simulink model "ELM_tictactoe_V2"  (R2021b)
settings: Solver=VariableStepAuto  StartTime=0.0  StopTime=inf  RelTol=1e-3
(part 2 of 136)

== system ELM_tictactoe_V2/Subsystem/Player Switcher a4 ==
  Key : Inport
  Switcher : Inport  Port=2
  AND 1 : MATLAB Function  TreatAsAtomicUnit=on
  Demultiplexer : Subsystem
      settings: PortSchema="{\"entries\":[{\"content\":{\"sides\":[{\"content\":{\"connectorIds\":[\"In1\"]},\"type\":\"ConnectorPlacement.EquallySpacedRectSide\",\"uuid\":\"6ccd7be5-9453-443a-8992-4f3046a94d81\"},{\"content\":{\"connectorIds\":[\"Out1\",\"Out2\"],\"side\":\"RIGHT\"},\"type\":\"ConnectorPlacement.EquallySpacedRectSide\",\"uuid\":\"9e3b2918-337b-479e-a737-e198b459be29\"},{\"content\":{\"connectorIds\":[],\"side\":\"TOP\"},\"type\":\"ConnectorPlacement.EquallySpacedRectSide\",\"uuid\":\"03b37edf-716a-49b3-8681-b476b437a461\"},{\"content\":{\"connectorIds\":[\"In2\"],\"side\":\"BOTTOM\"},\"type\":\"ConnectorPlacement.EquallySpacedRectSide\",\"uuid\":\"022ab476-2e55-4fe4-b85e-58af71f15e71\"}]},\"type\":\"ConnectorPlacement.EquallySpacedConnector\",\"uuid\":\"5541166b-b010-45a8-a1ab-2639d21d22e7\"}],\"packageUris\":[\"http://schema.mathworks.com/mf0/Connector/R2020b\"],\"version\":\"1.0\"}"
  Dlatch : Subsystem
  NOT : MATLAB Function  TreatAsAtomicUnit=on
  Unit Delay : UnitDelay  SampleTime=-1  HasFrameUpgradeWarning=on
  Unit Delay1 : UnitDelay  SampleTime=-1  HasFrameUpgradeWarning=on
  Unit Delay2 : UnitDelay  SampleTime=-1  HasFrameUpgradeWarning=on
  XOR5 : MATLAB Function  TreatAsAtomicUnit=on
  A : Outport
  B : Outport  Port=2
  wires:
  Key/1 -> Demultiplexer/1(Input), AND 1/1(input_a)
  Dlatch/1(Q) -> Demultiplexer/2(c)
  Demultiplexer/1(out0) -> XOR5/1(input_a), A/1
  Demultiplexer/2(out1) -> B/1, XOR5/2(input_b)
  Switcher/1 -> Dlatch/2(D)
  AND 1/1(output) -> Dlatch/1(Clock)  "o1"
  XOR5/1(output) -> NOT/1(input_a)  "o2"
  NOT/1(output) -> Unit Delay/1  "t1"
  Unit Delay/1 -> Unit Delay1/1
  Unit Delay1/1 -> Unit Delay2/1
  Unit Delay2/1 -> AND 1/2(input_b)

== system ELM_tictactoe_V2/Subsystem/Player Switcher a5 ==
  Key : Inport
  Switcher : Inport  Port=2
  AND 1 : MATLAB Function  TreatAsAtomicUnit=on
  Demultiplexer : Subsystem
      settings: PortSchema="{\"entries\":[{\"content\":{\"sides\":[{\"content\":{\"connectorIds\":[\"In1\"]},\"type\":\"ConnectorPlacement.EquallySpacedRectSide\",\"uuid\":\"6ccd7be5-9453-443a-8992-4f3046a94d81\"},{\"content\":{\"connectorIds\":[\"Out1\",\"Out2\"],\"side\":\"RIGHT\"},\"type\":\"ConnectorPlacement.EquallySpacedRectSide\",\"uuid\":\"9e3b2918-337b-479e-a737-e198b459be29\"},{\"content\":{\"connectorIds\":[],\"side\":\"TOP\"},\"type\":\"ConnectorPlacement.EquallySpacedRectSide\",\"uuid\":\"03b37edf-716a-49b3-8681-b476b437a461\"},{\"content\":{\"connectorIds\":[\"In2\"],\"side\":\"BOTTOM\"},\"type\":\"ConnectorPlacement.EquallySpacedRectSide\",\"uuid\":\"022ab476-2e55-4fe4-b85e-58af71f15e71\"}]},\"type\":\"ConnectorPlacement.EquallySpacedConnector\",\"uuid\":\"5541166b-b010-45a8-a1ab-2639d21d22e7\"}],\"packageUris\":[\"http://schema.mathworks.com/mf0/Connector/R2020b\"],\"version\":\"1.0\"}"
  Dlatch : Subsystem
  NOT : MATLAB Function  TreatAsAtomicUnit=on
  Unit Delay : UnitDelay  SampleTime=-1  HasFrameUpgradeWarning=on
  Unit Delay1 : UnitDelay  SampleTime=-1  HasFrameUpgradeWarning=on
  Unit Delay2 : UnitDelay  SampleTime=-1  HasFrameUpgradeWarning=on
  XOR5 : MATLAB Function  TreatAsAtomicUnit=on
  A : Outport
  B : Outport  Port=2
  wires:
  Key/1 -> Demultiplexer/1(Input), AND 1/1(input_a)
  Dlatch/1(Q) -> Demultiplexer/2(c)
  Demultiplexer/1(out0) -> XOR5/1(input_a), A/1
  Demultiplexer/2(out1) -> B/1, XOR5/2(input_b)
  Switcher/1 -> Dlatch/2(D)
  AND 1/1(output) -> Dlatch/1(Clock)  "o1"
  XOR5/1(output) -> NOT/1(input_a)  "o2"
  NOT/1(output) -> Unit Delay/1  "t1"
  Unit Delay/1 -> Unit Delay1/1
  Unit Delay1/1 -> Unit Delay2/1
  Unit Delay2/1 -> AND 1/2(input_b)

== system ELM_tictactoe_V2/Subsystem/Player Switcher a6 ==
  Key : Inport
  Switcher : Inport  Port=2
  AND 1 : MATLAB Function  TreatAsAtomicUnit=on
  Demultiplexer : Subsystem
      settings: PortSchema="{\"entries\":[{\"content\":{\"sides\":[{\"content\":{\"connectorIds\":[\"In1\"]},\"type\":\"ConnectorPlacement.EquallySpacedRectSide\",\"uuid\":\"6ccd7be5-9453-443a-8992-4f3046a94d81\"},{\"content\":{\"connectorIds\":[\"Out1\",\"Out2\"],\"side\":\"RIGHT\"},\"type\":\"ConnectorPlacement.EquallySpacedRectSide\",\"uuid\":\"9e3b2918-337b-479e-a737-e198b459be29\"},{\"content\":{\"connectorIds\":[],\"side\":\"TOP\"},\"type\":\"ConnectorPlacement.EquallySpacedRectSide\",\"uuid\":\"03b37edf-716a-49b3-8681-b476b437a461\"},{\"content\":{\"connectorIds\":[\"In2\"],\"side\":\"BOTTOM\"},\"type\":\"ConnectorPlacement.EquallySpacedRectSide\",\"uuid\":\"022ab476-2e55-4fe4-b85e-58af71f15e71\"}]},\"type\":\"ConnectorPlacement.EquallySpacedConnector\",\"uuid\":\"5541166b-b010-45a8-a1ab-2639d21d22e7\"}],\"packageUris\":[\"http://schema.mathworks.com/mf0/Connector/R2020b\"],\"version\":\"1.0\"}"
  Dlatch : Subsystem
  NOT : MATLAB Function  TreatAsAtomicUnit=on
  Unit Delay : UnitDelay  SampleTime=-1  HasFrameUpgradeWarning=on
  Unit Delay1 : UnitDelay  SampleTime=-1  HasFrameUpgradeWarning=on
  Unit Delay2 : UnitDelay  SampleTime=-1  HasFrameUpgradeWarning=on
  XOR5 : MATLAB Function  TreatAsAtomicUnit=on
  A : Outport
  B : Outport  Port=2
  wires:
  Key/1 -> Demultiplexer/1(Input), AND 1/1(input_a)
  Dlatch/1(Q) -> Demultiplexer/2(c)
  Demultiplexer/1(out0) -> XOR5/1(input_a), A/1
  Demultiplexer/2(out1) -> B/1, XOR5/2(input_b)
  Switcher/1 -> Dlatch/2(D)
  AND 1/1(output) -> Dlatch/1(Clock)  "o1"
  XOR5/1(output) -> NOT/1(input_a)  "o2"
  NOT/1(output) -> Unit Delay/1  "t1"
  Unit Delay/1 -> Unit Delay1/1
  Unit Delay1/1 -> Unit Delay2/1
  Unit Delay2/1 -> AND 1/2(input_b)

== system ELM_tictactoe_V2/Subsystem/Player Switcher a7 ==
  Key : Inport
  Switcher : Inport  Port=2
  AND 1 : MATLAB Function  TreatAsAtomicUnit=on
  Demultiplexer : Subsystem
      settings: PortSchema="{\"entries\":[{\"content\":{\"sides\":[{\"content\":{\"connectorIds\":[\"In1\"]},\"type\":\"ConnectorPlacement.EquallySpacedRectSide\",\"uuid\":\"6ccd7be5-9453-443a-8992-4f3046a94d81\"},{\"content\":{\"connectorIds\":[\"Out1\",\"Out2\"],\"side\":\"RIGHT\"},\"type\":\"ConnectorPlacement.EquallySpacedRectSide\",\"uuid\":\"9e3b2918-337b-479e-a737-e198b459be29\"},{\"content\":{\"connectorIds\":[],\"side\":\"TOP\"},\"type\":\"ConnectorPlacement.EquallySpacedRectSide\",\"uuid\":\"03b37edf-716a-49b3-8681-b476b437a461\"},{\"content\":{\"connectorIds\":[\"In2\"],\"side\":\"BOTTOM\"},\"type\":\"ConnectorPlacement.EquallySpacedRectSide\",\"uuid\":\"022ab476-2e55-4fe4-b85e-58af71f15e71\"}]},\"type\":\"ConnectorPlacement.EquallySpacedConnector\",\"uuid\":\"5541166b-b010-45a8-a1ab-2639d21d22e7\"}],\"packageUris\":[\"http://schema.mathworks.com/mf0/Connector/R2020b\"],\"version\":\"1.0\"}"
  Dlatch : Subsystem
  NOT : MATLAB Function  TreatAsAtomicUnit=on
  Unit Delay : UnitDelay  SampleTime=-1  HasFrameUpgradeWarning=on
  Unit Delay1 : UnitDelay  SampleTime=-1  HasFrameUpgradeWarning=on
  Unit Delay2 : UnitDelay  SampleTime=-1  HasFrameUpgradeWarning=on
  XOR5 : MATLAB Function  TreatAsAtomicUnit=on
  A : Outport
  B : Outport  Port=2
  wires:
  Key/1 -> Demultiplexer/1(Input), AND 1/1(input_a)
  Dlatch/1(Q) -> Demultiplexer/2(c)
  Demultiplexer/1(out0) -> XOR5/1(input_a), A/1
  Demultiplexer/2(out1) -> B/1, XOR5/2(input_b)
  Switcher/1 -> Dlatch/2(D)
  AND 1/1(output) -> Dlatch/1(Clock)  "o1"
  XOR5/1(output) -> NOT/1(input_a)  "o2"
  NOT/1(output) -> Unit Delay/1  "t1"
  Unit Delay/1 -> Unit Delay1/1
  Unit Delay1/1 -> Unit Delay2/1
  Unit Delay2/1 -> AND 1/2(input_b)

== system ELM_tictactoe_V2/Subsystem/Player Switcher a8 ==
  Key : Inport
  Switcher : Inport  Port=2
  AND 1 : MATLAB Function  TreatAsAtomicUnit=on
  Demultiplexer : Subsystem
      settings: PortSchema="{\"entries\":[{\"content\":{\"sides\":[{\"content\":{\"connectorIds\":[\"In1\"]},\"type\":\"ConnectorPlacement.EquallySpacedRectSide\",\"uuid\":\"6ccd7be5-9453-443a-8992-4f3046a94d81\"},{\"content\":{\"connectorIds\":[\"Out1\",\"Out2\"],\"side\":\"RIGHT\"},\"type\":\"ConnectorPlacement.EquallySpacedRectSide\",\"uuid\":\"9e3b2918-337b-479e-a737-e198b459be29\"},{\"content\":{\"connectorIds\":[],\"side\":\"TOP\"},\"type\":\"ConnectorPlacement.EquallySpacedRectSide\",\"uuid\":\"03b37edf-716a-49b3-8681-b476b437a461\"},{\"content\":{\"connectorIds\":[\"In2\"],\"side\":\"BOTTOM\"},\"type\":\"ConnectorPlacement.EquallySpacedRectSide\",\"uuid\":\"022ab476-2e55-4fe4-b85e-58af71f15e71\"}]},\"type\":\"ConnectorPlacement.EquallySpacedConnector\",\"uuid\":\"5541166b-b010-45a8-a1ab-2639d21d22e7\"}],\"packageUris\":[\"http://schema.mathworks.com/mf0/Connector/R2020b\"],\"version\":\"1.0\"}"
  Dlatch : Subsystem
  NOT : MATLAB Function  TreatAsAtomicUnit=on
  Unit Delay : UnitDelay  SampleTime=-1  HasFrameUpgradeWarning=on
  Unit Delay1 : UnitDelay  SampleTime=-1  HasFrameUpgradeWarning=on
  Unit Delay2 : UnitDelay  SampleTime=-1  HasFrameUpgradeWarning=on
  XOR5 : MATLAB Function  TreatAsAtomicUnit=on
  A : Outport
  B : Outport  Port=2
  wires:
  Key/1 -> Demultiplexer/1(Input), AND 1/1(input_a)
  Dlatch/1(Q) -> Demultiplexer/2(c)
  Demultiplexer/1(out0) -> XOR5/1(input_a), A/1
  Demultiplexer/2(out1) -> B/1, XOR5/2(input_b)
  Switcher/1 -> Dlatch/2(D)
  AND 1/1(output) -> Dlatch/1(Clock)  "o1"
  XOR5/1(output) -> NOT/1(input_a)  "o2"
  NOT/1(output) -> Unit Delay/1  "t1"
  Unit Delay/1 -> Unit Delay1/1
  Unit Delay1/1 -> Unit Delay2/1
  Unit Delay2/1 -> AND 1/2(input_b)

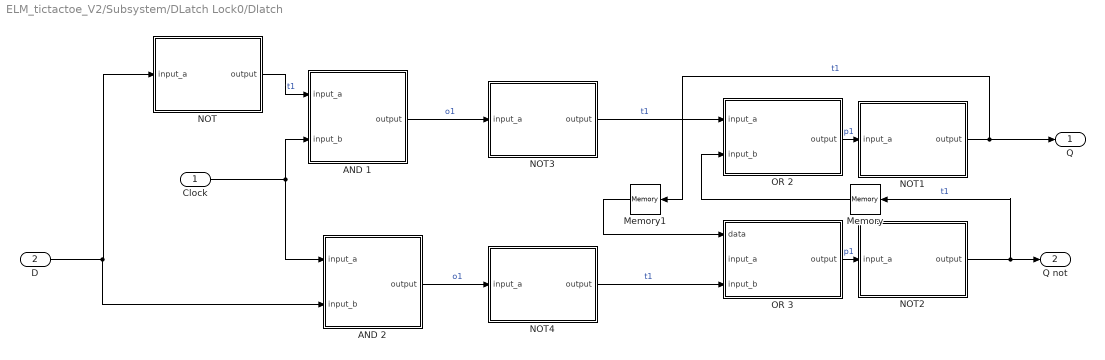
== system ELM_tictactoe_V2/Subsystem/DLatch Lock0/Dlatch ==
  Clock : Inport
  D : Inport  Port=2
  AND 1 : MATLAB Function  TreatAsAtomicUnit=on
  AND 2 : MATLAB Function  TreatAsAtomicUnit=on
  Memory : Memory
  Memory1 : Memory
  NOT : MATLAB Function  TreatAsAtomicUnit=on
  NOT1 : MATLAB Function  TreatAsAtomicUnit=on
  NOT2 : MATLAB Function  TreatAsAtomicUnit=on
  NOT3 : MATLAB Function  TreatAsAtomicUnit=on
  NOT4 : MATLAB Function  TreatAsAtomicUnit=on
  OR 2 : MATLAB Function  TreatAsAtomicUnit=on
  OR 3 : MATLAB Function  TreatAsAtomicUnit=on
  Q : Outport
  Q not : Outport  Port=2
  wires:
  D/1 -> AND 2/2(input_b), NOT/1(input_a)
  NOT/1(output) -> AND 1/1(input_a)  "t1"
  Clock/1 -> AND 1/2(input_b), AND 2/1(input_a)
  OR 2/1(output) -> NOT1/1(input_a)  "p1"
  OR 3/1(output) -> NOT2/1(input_a)  "p1"
  AND 2/1(output) -> NOT4/1(input_a)  "o1"
  NOT1/1(output) -> Q/1, Memory1/1  "t1"
  NOT2/1(output) -> Memory/1, Q not/1  "t1"
  AND 1/1(output) -> NOT3/1(input_a)  "o1"
  NOT3/1(output) -> OR 2/1(input_a)  "t1"
  NOT4/1(output) -> OR 3/3(input_b)  "t1"
  Memory/1 -> OR 2/2(input_b)
  Memory1/1 -> OR 3/1(data)

== system ELM_tictactoe_V2/Subsystem/DLatch Lock1/Dlatch ==
  D : Inport
  Clock : Inport  Port=2
  AND 1 : MATLAB Function  TreatAsAtomicUnit=on
  AND 2 : MATLAB Function  TreatAsAtomicUnit=on
  Memory : Memory  InitialCondition=1  LinearizeAsDelay=on
  Memory1 : Memory  LinearizeAsDelay=on
  NOT1 : MATLAB Function  TreatAsAtomicUnit=on
  NOT2 : MATLAB Function  TreatAsAtomicUnit=on
  NOT3 : MATLAB Function  TreatAsAtomicUnit=on
  OR 2 : MATLAB Function  TreatAsAtomicUnit=on
  OR 3 : MATLAB Function  TreatAsAtomicUnit=on
  Q : Outport
  Q not : Outport  Port=2
  wires:
  D/1 -> NOT3/1(input_a), AND 2/2(input_b)
  NOT3/1(output) -> AND 1/1(input_a)  "t1"
  Clock/1 -> AND 1/2(input_b), AND 2/1(input_a)
  OR 2/1(output) -> NOT1/1(input_a)  "p1"
  OR 3/1(output) -> NOT2/1(input_a)  "p1"
  AND 2/1(output) -> OR 3/2(input_b)  "o1"
  NOT1/1(output) -> Memory1/1, Q/1  "t1"
  NOT2/1(output) -> Memory/1, Q not/1  "t1"
  AND 1/1(output) -> OR 2/1(input_a)  "t1"
  Memory/1 -> OR 2/2(input_b)
  Memory1/1 -> OR 3/1(input_a)

== system ELM_tictactoe_V2/Subsystem/DLatch Lock2/Dlatch ==
  D : Inport
  Clock : Inport  Port=2
  AND 1 : MATLAB Function  TreatAsAtomicUnit=on
  AND 2 : MATLAB Function  TreatAsAtomicUnit=on
  Memory : Memory  InitialCondition=1  LinearizeAsDelay=on
  Memory1 : Memory  LinearizeAsDelay=on
  NOT1 : MATLAB Function  TreatAsAtomicUnit=on
  NOT2 : MATLAB Function  TreatAsAtomicUnit=on
  NOT3 : MATLAB Function  TreatAsAtomicUnit=on
  OR 2 : MATLAB Function  TreatAsAtomicUnit=on
  OR 3 : MATLAB Function  TreatAsAtomicUnit=on
  Q : Outport
  Q not : Outport  Port=2
  wires:
  D/1 -> NOT3/1(input_a), AND 2/2(input_b)
  NOT3/1(output) -> AND 1/1(input_a)  "t1"
  Clock/1 -> AND 1/2(input_b), AND 2/1(input_a)
  OR 2/1(output) -> NOT1/1(input_a)  "p1"
  OR 3/1(output) -> NOT2/1(input_a)  "p1"
  AND 2/1(output) -> OR 3/2(input_b)  "o1"
  NOT1/1(output) -> Memory1/1, Q/1  "t1"
  NOT2/1(output) -> Memory/1, Q not/1  "t1"
  AND 1/1(output) -> OR 2/1(input_a)  "t1"
  Memory/1 -> OR 2/2(input_b)
  Memory1/1 -> OR 3/1(input_a)

== system ELM_tictactoe_V2/Subsystem/DLatch Lock3/Dlatch ==
  D : Inport
  Clock : Inport  Port=2
  AND 1 : MATLAB Function  TreatAsAtomicUnit=on
  AND 2 : MATLAB Function  TreatAsAtomicUnit=on
  Memory : Memory  InitialCondition=1  LinearizeAsDelay=on
  Memory1 : Memory  LinearizeAsDelay=on
  NOT1 : MATLAB Function  TreatAsAtomicUnit=on
  NOT2 : MATLAB Function  TreatAsAtomicUnit=on
  NOT3 : MATLAB Function  TreatAsAtomicUnit=on
  OR 2 : MATLAB Function  TreatAsAtomicUnit=on
  OR 3 : MATLAB Function  TreatAsAtomicUnit=on
  Q : Outport
  Q not : Outport  Port=2
  wires:
  D/1 -> NOT3/1(input_a), AND 2/2(input_b)
  NOT3/1(output) -> AND 1/1(input_a)  "t1"
  Clock/1 -> AND 1/2(input_b), AND 2/1(input_a)
  OR 2/1(output) -> NOT1/1(input_a)  "p1"
  OR 3/1(output) -> NOT2/1(input_a)  "p1"
  AND 2/1(output) -> OR 3/2(input_b)  "o1"
  NOT1/1(output) -> Memory1/1, Q/1  "t1"
  NOT2/1(output) -> Memory/1, Q not/1  "t1"
  AND 1/1(output) -> OR 2/1(input_a)  "t1"
  Memory/1 -> OR 2/2(input_b)
  Memory1/1 -> OR 3/1(input_a)

== system ELM_tictactoe_V2/Subsystem/DLatch Lock4/Dlatch ==
  D : Inport
  Clock : Inport  Port=2
  AND 1 : MATLAB Function  TreatAsAtomicUnit=on
  AND 2 : MATLAB Function  TreatAsAtomicUnit=on
  Memory : Memory  InitialCondition=1  LinearizeAsDelay=on
  Memory1 : Memory  LinearizeAsDelay=on
  NOT1 : MATLAB Function  TreatAsAtomicUnit=on
  NOT2 : MATLAB Function  TreatAsAtomicUnit=on
  NOT3 : MATLAB Function  TreatAsAtomicUnit=on
  OR 2 : MATLAB Function  TreatAsAtomicUnit=on
  OR 3 : MATLAB Function  TreatAsAtomicUnit=on
  Q : Outport
  Q not : Outport  Port=2
  wires:
  D/1 -> NOT3/1(input_a), AND 2/2(input_b)
  NOT3/1(output) -> AND 1/1(input_a)  "t1"
  Clock/1 -> AND 1/2(input_b), AND 2/1(input_a)
  OR 2/1(output) -> NOT1/1(input_a)  "p1"
  OR 3/1(output) -> NOT2/1(input_a)  "p1"
  AND 2/1(output) -> OR 3/2(input_b)  "o1"
  NOT1/1(output) -> Memory1/1, Q/1  "t1"
  NOT2/1(output) -> Memory/1, Q not/1  "t1"
  AND 1/1(output) -> OR 2/1(input_a)  "t1"
  Memory/1 -> OR 2/2(input_b)
  Memory1/1 -> OR 3/1(input_a)

== system ELM_tictactoe_V2/Subsystem/DLatch Lock5/Dlatch ==
  D : Inport
  Clock : Inport  Port=2
  AND 1 : MATLAB Function  TreatAsAtomicUnit=on
  AND 2 : MATLAB Function  TreatAsAtomicUnit=on
  Memory : Memory  InitialCondition=1  LinearizeAsDelay=on
  Memory1 : Memory  LinearizeAsDelay=on
  NOT1 : MATLAB Function  TreatAsAtomicUnit=on
  NOT2 : MATLAB Function  TreatAsAtomicUnit=on
  NOT3 : MATLAB Function  TreatAsAtomicUnit=on
  OR 2 : MATLAB Function  TreatAsAtomicUnit=on
  OR 3 : MATLAB Function  TreatAsAtomicUnit=on
  Q : Outport
  Q not : Outport  Port=2
  wires:
  D/1 -> NOT3/1(input_a), AND 2/2(input_b)
  NOT3/1(output) -> AND 1/1(input_a)  "t1"
  Clock/1 -> AND 1/2(input_b), AND 2/1(input_a)
  OR 2/1(output) -> NOT1/1(input_a)  "p1"
  OR 3/1(output) -> NOT2/1(input_a)  "p1"
  AND 2/1(output) -> OR 3/2(input_b)  "o1"
  NOT1/1(output) -> Memory1/1, Q/1  "t1"
  NOT2/1(output) -> Memory/1, Q not/1  "t1"
  AND 1/1(output) -> OR 2/1(input_a)  "t1"
  Memory/1 -> OR 2/2(input_b)
  Memory1/1 -> OR 3/1(input_a)

== system ELM_tictactoe_V2/Subsystem/DLatch Lock6/Dlatch ==
  D : Inport
  Clock : Inport  Port=2
  AND 1 : MATLAB Function  TreatAsAtomicUnit=on
  AND 2 : MATLAB Function  TreatAsAtomicUnit=on
  Memory : Memory  InitialCondition=1  LinearizeAsDelay=on
  Memory1 : Memory  LinearizeAsDelay=on
  NOT1 : MATLAB Function  TreatAsAtomicUnit=on
  NOT2 : MATLAB Function  TreatAsAtomicUnit=on
  NOT3 : MATLAB Function  TreatAsAtomicUnit=on
  OR 2 : MATLAB Function  TreatAsAtomicUnit=on
  OR 3 : MATLAB Function  TreatAsAtomicUnit=on
  Q : Outport
  Q not : Outport  Port=2
  wires:
  D/1 -> NOT3/1(input_a), AND 2/2(input_b)
  NOT3/1(output) -> AND 1/1(input_a)  "t1"
  Clock/1 -> AND 1/2(input_b), AND 2/1(input_a)
  OR 2/1(output) -> NOT1/1(input_a)  "p1"
  OR 3/1(output) -> NOT2/1(input_a)  "p1"
  AND 2/1(output) -> OR 3/2(input_b)  "o1"
  NOT1/1(output) -> Memory1/1, Q/1  "t1"
  NOT2/1(output) -> Memory/1, Q not/1  "t1"
  AND 1/1(output) -> OR 2/1(input_a)  "t1"
  Memory/1 -> OR 2/2(input_b)
  Memory1/1 -> OR 3/1(input_a)

== system ELM_tictactoe_V2/Subsystem/DLatch Lock7/Dlatch ==
  D : Inport
  Clock : Inport  Port=2
  AND 1 : MATLAB Function  TreatAsAtomicUnit=on
  AND 2 : MATLAB Function  TreatAsAtomicUnit=on
  Memory : Memory  InitialCondition=1  LinearizeAsDelay=on
  Memory1 : Memory  LinearizeAsDelay=on
  NOT1 : MATLAB Function  TreatAsAtomicUnit=on
  NOT2 : MATLAB Function  TreatAsAtomicUnit=on
  NOT3 : MATLAB Function  TreatAsAtomicUnit=on
  OR 2 : MATLAB Function  TreatAsAtomicUnit=on
  OR 3 : MATLAB Function  TreatAsAtomicUnit=on
  Q : Outport
  Q not : Outport  Port=2
  wires:
  D/1 -> NOT3/1(input_a), AND 2/2(input_b)
  NOT3/1(output) -> AND 1/1(input_a)  "t1"
  Clock/1 -> AND 1/2(input_b), AND 2/1(input_a)
  OR 2/1(output) -> NOT1/1(input_a)  "p1"
  OR 3/1(output) -> NOT2/1(input_a)  "p1"
  AND 2/1(output) -> OR 3/2(input_b)  "o1"
  NOT1/1(output) -> Memory1/1, Q/1  "t1"
  NOT2/1(output) -> Memory/1, Q not/1  "t1"
  AND 1/1(output) -> OR 2/1(input_a)  "t1"
  Memory/1 -> OR 2/2(input_b)
  Memory1/1 -> OR 3/1(input_a)

== system ELM_tictactoe_V2/Subsystem/DLatch Lock8/Dlatch ==
  D : Inport
  Clock : Inport  Port=2
  AND 1 : MATLAB Function  TreatAsAtomicUnit=on
  AND 2 : MATLAB Function  TreatAsAtomicUnit=on
  Memory : Memory  InitialCondition=1  LinearizeAsDelay=on
  Memory1 : Memory  LinearizeAsDelay=on
  NOT1 : MATLAB Function  TreatAsAtomicUnit=on
  NOT2 : MATLAB Function  TreatAsAtomicUnit=on
  NOT3 : MATLAB Function  TreatAsAtomicUnit=on
  OR 2 : MATLAB Function  TreatAsAtomicUnit=on
  OR 3 : MATLAB Function  TreatAsAtomicUnit=on
  Q : Outport
  Q not : Outport  Port=2
  wires:
  D/1 -> NOT3/1(input_a), AND 2/2(input_b)
  NOT3/1(output) -> AND 1/1(input_a)  "t1"
  Clock/1 -> AND 1/2(input_b), AND 2/1(input_a)
  OR 2/1(output) -> NOT1/1(input_a)  "p1"
  OR 3/1(output) -> NOT2/1(input_a)  "p1"
  AND 2/1(output) -> OR 3/2(input_b)  "o1"
  NOT1/1(output) -> Memory1/1, Q/1  "t1"
  NOT2/1(output) -> Memory/1, Q not/1  "t1"
  AND 1/1(output) -> OR 2/1(input_a)  "t1"
  Memory/1 -> OR 2/2(input_b)
  Memory1/1 -> OR 3/1(input_a)

== system ELM_tictactoe_V2/Subsystem/DLatch Lock9/Dlatch ==
  D : Inport
  Clock : Inport  Port=2
  AND 1 : MATLAB Function  TreatAsAtomicUnit=on
  AND 2 : MATLAB Function  TreatAsAtomicUnit=on
  Memory : Memory  InitialCondition=1  LinearizeAsDelay=on
  Memory1 : Memory  LinearizeAsDelay=on
  NOT1 : MATLAB Function  TreatAsAtomicUnit=on
  NOT2 : MATLAB Function  TreatAsAtomicUnit=on
  NOT3 : MATLAB Function  TreatAsAtomicUnit=on
  OR 2 : MATLAB Function  TreatAsAtomicUnit=on
  OR 3 : MATLAB Function  TreatAsAtomicUnit=on
  Q : Outport
  Q not : Outport  Port=2
  wires:
  D/1 -> NOT3/1(input_a), AND 2/2(input_b)
  NOT3/1(output) -> AND 1/1(input_a)  "t1"
  Clock/1 -> AND 1/2(input_b), AND 2/1(input_a)
  OR 2/1(output) -> NOT1/1(input_a)  "p1"
  OR 3/1(output) -> NOT2/1(input_a)  "p1"
  AND 2/1(output) -> OR 3/2(input_b)  "o1"
  NOT1/1(output) -> Memory1/1, Q/1  "t1"
  NOT2/1(output) -> Memory/1, Q not/1  "t1"
  AND 1/1(output) -> OR 2/1(input_a)  "t1"
  Memory/1 -> OR 2/2(input_b)
  Memory1/1 -> OR 3/1(input_a)

== system ELM_tictactoe_V2/Subsystem/Player Switcher a/Demultiplexer ==
  note: if problems switch outputs
  Input : Inport
  c : Inport  Port=2
  AND 1 : MATLAB Function  TreatAsAtomicUnit=on
  AND 2 : MATLAB Function  TreatAsAtomicUnit=on
  NOT : MATLAB Function  TreatAsAtomicUnit=on
  out0 : Outport
  out1 : Outport  Port=2
  wires:
  c/1 -> AND 1/2(input_b), NOT/1(input_a)
  AND 2/1(output) -> out0/1  "o1"
  AND 1/1(output) -> out1/1  "o1"
  Input/1 -> AND 1/1(input_a), AND 2/2(input_b)
  NOT/1(output) -> AND 2/1(input_a)  "t1"

== system ELM_tictactoe_V2/Subsystem/Player Switcher a/Dlatch ==
  Clock : Inport
  D : Inport  Port=2
  AND 1 : MATLAB Function  TreatAsAtomicUnit=on
  AND 2 : MATLAB Function  TreatAsAtomicUnit=on
  Memory : Memory  InitialCondition=1  LinearizeAsDelay=on
  Memory1 : Memory  LinearizeAsDelay=on
  NOT : MATLAB Function  TreatAsAtomicUnit=on
  NOT1 : MATLAB Function  TreatAsAtomicUnit=on
  NOT2 : MATLAB Function  TreatAsAtomicUnit=on
  OR 2 : MATLAB Function  TreatAsAtomicUnit=on
  OR 3 : MATLAB Function  TreatAsAtomicUnit=on
  Q : Outport
  Q not : Outport  Port=2
  wires:
  D/1 -> AND 2/2(input_b), NOT/1(input_a)
  NOT/1(output) -> AND 1/1(input_a)  "t1"
  Clock/1 -> AND 1/2(input_b), AND 2/1(input_a)
  OR 2/1(output) -> NOT1/1(input_a)  "p1"
  OR 3/1(output) -> NOT2/1(input_a)  "p1"
  AND 2/1(output) -> OR 3/2(input_b)  "o1"
  NOT1/1(output) -> Memory1/1, Q/1  "t1"
  NOT2/1(output) -> Memory/1, Q not/1  "t1"
  AND 1/1(output) -> OR 2/1(input_a)  "t1"
  Memory/1 -> OR 2/2(input_b)
  Memory1/1 -> OR 3/1(input_a)

== system ELM_tictactoe_V2/Subsystem/Player Switcher a1/Demultiplexer ==
  note: if problems switch outputs
  Input : Inport
  c : Inport  Port=2
  AND 1 : MATLAB Function  TreatAsAtomicUnit=on
  AND 2 : MATLAB Function  TreatAsAtomicUnit=on
  NOT : MATLAB Function  TreatAsAtomicUnit=on
  out0 : Outport
  out1 : Outport  Port=2
  wires:
  c/1 -> AND 1/2(input_b), NOT/1(input_a)
  AND 2/1(output) -> out0/1  "o1"
  AND 1/1(output) -> out1/1  "o1"
  Input/1 -> AND 1/1(input_a), AND 2/2(input_b)
  NOT/1(output) -> AND 2/1(input_a)  "t1"

== system ELM_tictactoe_V2/Subsystem/Player Switcher a1/Dlatch ==
  Clock : Inport
  D : Inport  Port=2
  AND 1 : MATLAB Function  TreatAsAtomicUnit=on
  AND 2 : MATLAB Function  TreatAsAtomicUnit=on
  Memory : Memory  InitialCondition=1  LinearizeAsDelay=on
  Memory1 : Memory  LinearizeAsDelay=on
  NOT : MATLAB Function  TreatAsAtomicUnit=on
  NOT1 : MATLAB Function  TreatAsAtomicUnit=on
  NOT2 : MATLAB Function  TreatAsAtomicUnit=on
  OR 2 : MATLAB Function  TreatAsAtomicUnit=on
  OR 3 : MATLAB Function  TreatAsAtomicUnit=on
  Q : Outport
  Q not : Outport  Port=2
  wires:
  D/1 -> AND 2/2(input_b), NOT/1(input_a)
  NOT/1(output) -> AND 1/1(input_a)  "t1"
  Clock/1 -> AND 1/2(input_b), AND 2/1(input_a)
  OR 2/1(output) -> NOT1/1(input_a)  "p1"
  OR 3/1(output) -> NOT2/1(input_a)  "p1"
  AND 2/1(output) -> OR 3/2(input_b)  "o1"
  NOT1/1(output) -> Memory1/1, Q/1  "t1"
  NOT2/1(output) -> Memory/1, Q not/1  "t1"
  AND 1/1(output) -> OR 2/1(input_a)  "t1"
  Memory/1 -> OR 2/2(input_b)
  Memory1/1 -> OR 3/1(input_a)

== system ELM_tictactoe_V2/Subsystem/Player Switcher a2/Demultiplexer ==
  note: if problems switch outputs
  Input : Inport
  c : Inport  Port=2
  AND 1 : MATLAB Function  TreatAsAtomicUnit=on
  AND 2 : MATLAB Function  TreatAsAtomicUnit=on
  NOT : MATLAB Function  TreatAsAtomicUnit=on
  out0 : Outport
  out1 : Outport  Port=2
  wires:
  c/1 -> AND 1/2(input_b), NOT/1(input_a)
  AND 2/1(output) -> out0/1  "o1"
  AND 1/1(output) -> out1/1  "o1"
  Input/1 -> AND 1/1(input_a), AND 2/2(input_b)
  NOT/1(output) -> AND 2/1(input_a)  "t1"

== system ELM_tictactoe_V2/Subsystem/Player Switcher a2/Dlatch ==
  Clock : Inport
  D : Inport  Port=2
  AND 1 : MATLAB Function  TreatAsAtomicUnit=on
  AND 2 : MATLAB Function  TreatAsAtomicUnit=on
  Memory : Memory  InitialCondition=1  LinearizeAsDelay=on
  Memory1 : Memory  LinearizeAsDelay=on
  NOT : MATLAB Function  TreatAsAtomicUnit=on
  NOT1 : MATLAB Function  TreatAsAtomicUnit=on
  NOT2 : MATLAB Function  TreatAsAtomicUnit=on
  OR 2 : MATLAB Function  TreatAsAtomicUnit=on
  OR 3 : MATLAB Function  TreatAsAtomicUnit=on
  Q : Outport
  Q not : Outport  Port=2
  wires:
  D/1 -> AND 2/2(input_b), NOT/1(input_a)
  NOT/1(output) -> AND 1/1(input_a)  "t1"
  Clock/1 -> AND 1/2(input_b), AND 2/1(input_a)
  OR 2/1(output) -> NOT1/1(input_a)  "p1"
  OR 3/1(output) -> NOT2/1(input_a)  "p1"
  AND 2/1(output) -> OR 3/2(input_b)  "o1"
  NOT1/1(output) -> Memory1/1, Q/1  "t1"
  NOT2/1(output) -> Memory/1, Q not/1  "t1"
  AND 1/1(output) -> OR 2/1(input_a)  "t1"
  Memory/1 -> OR 2/2(input_b)
  Memory1/1 -> OR 3/1(input_a)

== system ELM_tictactoe_V2/Subsystem/Player Switcher a3/Demultiplexer ==
  note: if problems switch outputs
  Input : Inport
  c : Inport  Port=2
  AND 1 : MATLAB Function  TreatAsAtomicUnit=on
  AND 2 : MATLAB Function  TreatAsAtomicUnit=on
  NOT : MATLAB Function  TreatAsAtomicUnit=on
  out0 : Outport
  out1 : Outport  Port=2
  wires:
  c/1 -> AND 1/2(input_b), NOT/1(input_a)
  AND 2/1(output) -> out0/1  "o1"
  AND 1/1(output) -> out1/1  "o1"
  Input/1 -> AND 1/1(input_a), AND 2/2(input_b)
  NOT/1(output) -> AND 2/1(input_a)  "t1"

== system ELM_tictactoe_V2/Subsystem/Player Switcher a3/Dlatch ==
  Clock : Inport
  D : Inport  Port=2
  AND 1 : MATLAB Function  TreatAsAtomicUnit=on
  AND 2 : MATLAB Function  TreatAsAtomicUnit=on
  Memory : Memory  InitialCondition=1  LinearizeAsDelay=on
  Memory1 : Memory  LinearizeAsDelay=on
  NOT : MATLAB Function  TreatAsAtomicUnit=on
  NOT1 : MATLAB Function  TreatAsAtomicUnit=on
  NOT2 : MATLAB Function  TreatAsAtomicUnit=on
  OR 2 : MATLAB Function  TreatAsAtomicUnit=on
  OR 3 : MATLAB Function  TreatAsAtomicUnit=on
  Q : Outport
  Q not : Outport  Port=2
  wires:
  D/1 -> AND 2/2(input_b), NOT/1(input_a)
  NOT/1(output) -> AND 1/1(input_a)  "t1"
  Clock/1 -> AND 1/2(input_b), AND 2/1(input_a)
  OR 2/1(output) -> NOT1/1(input_a)  "p1"
  OR 3/1(output) -> NOT2/1(input_a)  "p1"
  AND 2/1(output) -> OR 3/2(input_b)  "o1"
  NOT1/1(output) -> Memory1/1, Q/1  "t1"
  NOT2/1(output) -> Memory/1, Q not/1  "t1"
  AND 1/1(output) -> OR 2/1(input_a)  "t1"
  Memory/1 -> OR 2/2(input_b)
  Memory1/1 -> OR 3/1(input_a)

== system ELM_tictactoe_V2/Subsystem/Player Switcher a4/Demultiplexer ==
  note: if problems switch outputs
  Input : Inport
  c : Inport  Port=2
  AND 1 : MATLAB Function  TreatAsAtomicUnit=on
  AND 2 : MATLAB Function  TreatAsAtomicUnit=on
  NOT : MATLAB Function  TreatAsAtomicUnit=on
  out0 : Outport
  out1 : Outport  Port=2
  wires:
  c/1 -> AND 1/2(input_b), NOT/1(input_a)
  AND 2/1(output) -> out0/1  "o1"
  AND 1/1(output) -> out1/1  "o1"
  Input/1 -> AND 1/1(input_a), AND 2/2(input_b)
  NOT/1(output) -> AND 2/1(input_a)  "t1"

== system ELM_tictactoe_V2/Subsystem/Player Switcher a4/Dlatch ==
  Clock : Inport
  D : Inport  Port=2
  AND 1 : MATLAB Function  TreatAsAtomicUnit=on
  AND 2 : MATLAB Function  TreatAsAtomicUnit=on
  Memory : Memory  InitialCondition=1  LinearizeAsDelay=on
  Memory1 : Memory  LinearizeAsDelay=on
  NOT : MATLAB Function  TreatAsAtomicUnit=on
  NOT1 : MATLAB Function  TreatAsAtomicUnit=on
  NOT2 : MATLAB Function  TreatAsAtomicUnit=on
  OR 2 : MATLAB Function  TreatAsAtomicUnit=on
  OR 3 : MATLAB Function  TreatAsAtomicUnit=on
  Q : Outport
  Q not : Outport  Port=2
  wires:
  D/1 -> AND 2/2(input_b), NOT/1(input_a)
  NOT/1(output) -> AND 1/1(input_a)  "t1"
  Clock/1 -> AND 1/2(input_b), AND 2/1(input_a)
  OR 2/1(output) -> NOT1/1(input_a)  "p1"
  OR 3/1(output) -> NOT2/1(input_a)  "p1"
  AND 2/1(output) -> OR 3/2(input_b)  "o1"
  NOT1/1(output) -> Memory1/1, Q/1  "t1"
  NOT2/1(output) -> Memory/1, Q not/1  "t1"
  AND 1/1(output) -> OR 2/1(input_a)  "t1"
  Memory/1 -> OR 2/2(input_b)
  Memory1/1 -> OR 3/1(input_a)

== system ELM_tictactoe_V2/Subsystem/Player Switcher a5/Demultiplexer ==
  note: if problems switch outputs
  Input : Inport
  c : Inport  Port=2
  AND 1 : MATLAB Function  TreatAsAtomicUnit=on
  AND 2 : MATLAB Function  TreatAsAtomicUnit=on
  NOT : MATLAB Function  TreatAsAtomicUnit=on
  out0 : Outport
  out1 : Outport  Port=2
  wires:
  c/1 -> AND 1/2(input_b), NOT/1(input_a)
  AND 2/1(output) -> out0/1  "o1"
  AND 1/1(output) -> out1/1  "o1"
  Input/1 -> AND 1/1(input_a), AND 2/2(input_b)
  NOT/1(output) -> AND 2/1(input_a)  "t1"

== system ELM_tictactoe_V2/Subsystem/Player Switcher a5/Dlatch ==
  Clock : Inport
  D : Inport  Port=2
  AND 1 : MATLAB Function  TreatAsAtomicUnit=on
  AND 2 : MATLAB Function  TreatAsAtomicUnit=on
  Memory : Memory  InitialCondition=1  LinearizeAsDelay=on
  Memory1 : Memory  LinearizeAsDelay=on
  NOT : MATLAB Function  TreatAsAtomicUnit=on
  NOT1 : MATLAB Function  TreatAsAtomicUnit=on
  NOT2 : MATLAB Function  TreatAsAtomicUnit=on
  OR 2 : MATLAB Function  TreatAsAtomicUnit=on
  OR 3 : MATLAB Function  TreatAsAtomicUnit=on
  Q : Outport
  Q not : Outport  Port=2
  wires:
  D/1 -> AND 2/2(input_b), NOT/1(input_a)
  NOT/1(output) -> AND 1/1(input_a)  "t1"
  Clock/1 -> AND 1/2(input_b), AND 2/1(input_a)
  OR 2/1(output) -> NOT1/1(input_a)  "p1"
  OR 3/1(output) -> NOT2/1(input_a)  "p1"
  AND 2/1(output) -> OR 3/2(input_b)  "o1"
  NOT1/1(output) -> Memory1/1, Q/1  "t1"
  NOT2/1(output) -> Memory/1, Q not/1  "t1"
  AND 1/1(output) -> OR 2/1(input_a)  "t1"
  Memory/1 -> OR 2/2(input_b)
  Memory1/1 -> OR 3/1(input_a)

== system ELM_tictactoe_V2/Subsystem/Player Switcher a6/Demultiplexer ==
  note: if problems switch outputs
  Input : Inport
  c : Inport  Port=2
  AND 1 : MATLAB Function  TreatAsAtomicUnit=on
  AND 2 : MATLAB Function  TreatAsAtomicUnit=on
  NOT : MATLAB Function  TreatAsAtomicUnit=on
  out0 : Outport
  out1 : Outport  Port=2
  wires:
  c/1 -> AND 1/2(input_b), NOT/1(input_a)
  AND 2/1(output) -> out0/1  "o1"
  AND 1/1(output) -> out1/1  "o1"
  Input/1 -> AND 1/1(input_a), AND 2/2(input_b)
  NOT/1(output) -> AND 2/1(input_a)  "t1"

== system ELM_tictactoe_V2/Subsystem/Player Switcher a6/Dlatch ==
  Clock : Inport
  D : Inport  Port=2
  AND 1 : MATLAB Function  TreatAsAtomicUnit=on
  AND 2 : MATLAB Function  TreatAsAtomicUnit=on
  Memory : Memory  InitialCondition=1  LinearizeAsDelay=on
  Memory1 : Memory  LinearizeAsDelay=on
  NOT : MATLAB Function  TreatAsAtomicUnit=on
  NOT1 : MATLAB Function  TreatAsAtomicUnit=on
  NOT2 : MATLAB Function  TreatAsAtomicUnit=on
  OR 2 : MATLAB Function  TreatAsAtomicUnit=on
  OR 3 : MATLAB Function  TreatAsAtomicUnit=on
  Q : Outport
  Q not : Outport  Port=2
  wires:
  D/1 -> AND 2/2(input_b), NOT/1(input_a)
  NOT/1(output) -> AND 1/1(input_a)  "t1"
  Clock/1 -> AND 1/2(input_b), AND 2/1(input_a)
  OR 2/1(output) -> NOT1/1(input_a)  "p1"
  OR 3/1(output) -> NOT2/1(input_a)  "p1"
  AND 2/1(output) -> OR 3/2(input_b)  "o1"
  NOT1/1(output) -> Memory1/1, Q/1  "t1"
  NOT2/1(output) -> Memory/1, Q not/1  "t1"
  AND 1/1(output) -> OR 2/1(input_a)  "t1"
  Memory/1 -> OR 2/2(input_b)
  Memory1/1 -> OR 3/1(input_a)

== system ELM_tictactoe_V2/Subsystem/Player Switcher a7/Demultiplexer ==
  note: if problems switch outputs
  Input : Inport
  c : Inport  Port=2
  AND 1 : MATLAB Function  TreatAsAtomicUnit=on
  AND 2 : MATLAB Function  TreatAsAtomicUnit=on
  NOT : MATLAB Function  TreatAsAtomicUnit=on
  out0 : Outport
  out1 : Outport  Port=2
  wires:
  c/1 -> AND 1/2(input_b), NOT/1(input_a)
  AND 2/1(output) -> out0/1  "o1"
  AND 1/1(output) -> out1/1  "o1"
  Input/1 -> AND 1/1(input_a), AND 2/2(input_b)
  NOT/1(output) -> AND 2/1(input_a)  "t1"

== system ELM_tictactoe_V2/Subsystem/Player Switcher a7/Dlatch ==
  Clock : Inport
  D : Inport  Port=2
  AND 1 : MATLAB Function  TreatAsAtomicUnit=on
  AND 2 : MATLAB Function  TreatAsAtomicUnit=on
  Memory : Memory  InitialCondition=1  LinearizeAsDelay=on
  Memory1 : Memory  LinearizeAsDelay=on
  NOT : MATLAB Function  TreatAsAtomicUnit=on
  NOT1 : MATLAB Function  TreatAsAtomicUnit=on
  NOT2 : MATLAB Function  TreatAsAtomicUnit=on
  OR 2 : MATLAB Function  TreatAsAtomicUnit=on
  OR 3 : MATLAB Function  TreatAsAtomicUnit=on
  Q : Outport
  Q not : Outport  Port=2
  wires:
  D/1 -> AND 2/2(input_b), NOT/1(input_a)
  NOT/1(output) -> AND 1/1(input_a)  "t1"
  Clock/1 -> AND 1/2(input_b), AND 2/1(input_a)
  OR 2/1(output) -> NOT1/1(input_a)  "p1"
  OR 3/1(output) -> NOT2/1(input_a)  "p1"
  AND 2/1(output) -> OR 3/2(input_b)  "o1"
  NOT1/1(output) -> Memory1/1, Q/1  "t1"
  NOT2/1(output) -> Memory/1, Q not/1  "t1"
  AND 1/1(output) -> OR 2/1(input_a)  "t1"
  Memory/1 -> OR 2/2(input_b)
  Memory1/1 -> OR 3/1(input_a)

== system ELM_tictactoe_V2/Subsystem/Player Switcher a8/Demultiplexer ==
  note: if problems switch outputs
  Input : Inport
  c : Inport  Port=2
  AND 1 : MATLAB Function  TreatAsAtomicUnit=on
  AND 2 : MATLAB Function  TreatAsAtomicUnit=on
  NOT : MATLAB Function  TreatAsAtomicUnit=on
  out0 : Outport
  out1 : Outport  Port=2
  wires:
  c/1 -> AND 1/2(input_b), NOT/1(input_a)
  AND 2/1(output) -> out0/1  "o1"
  AND 1/1(output) -> out1/1  "o1"
  Input/1 -> AND 1/1(input_a), AND 2/2(input_b)
  NOT/1(output) -> AND 2/1(input_a)  "t1"

== system ELM_tictactoe_V2/Subsystem/Player Switcher a8/Dlatch ==
  Clock : Inport
  D : Inport  Port=2
  AND 1 : MATLAB Function  TreatAsAtomicUnit=on
  AND 2 : MATLAB Function  TreatAsAtomicUnit=on
  Memory : Memory  InitialCondition=1  LinearizeAsDelay=on
  Memory1 : Memory  LinearizeAsDelay=on
  NOT : MATLAB Function  TreatAsAtomicUnit=on
  NOT1 : MATLAB Function  TreatAsAtomicUnit=on
  NOT2 : MATLAB Function  TreatAsAtomicUnit=on
  OR 2 : MATLAB Function  TreatAsAtomicUnit=on
  OR 3 : MATLAB Function  TreatAsAtomicUnit=on
  Q : Outport
  Q not : Outport  Port=2
  wires:
  D/1 -> AND 2/2(input_b), NOT/1(input_a)
  NOT/1(output) -> AND 1/1(input_a)  "t1"
  Clock/1 -> AND 1/2(input_b), AND 2/1(input_a)
  OR 2/1(output) -> NOT1/1(input_a)  "p1"
  OR 3/1(output) -> NOT2/1(input_a)  "p1"
  AND 2/1(output) -> OR 3/2(input_b)  "o1"
  NOT1/1(output) -> Memory1/1, Q/1  "t1"
  NOT2/1(output) -> Memory/1, Q not/1  "t1"
  AND 1/1(output) -> OR 2/1(input_a)  "t1"
  Memory/1 -> OR 2/2(input_b)
  Memory1/1 -> OR 3/1(input_a)

== matlab function ELM_tictactoe_V2/Subsystem/Player Switcher a3/AND 1 ==
  data: input_a input; output output; input_b input
function output = ELM_AND_GATE(input_a,input_b)

W_in = [-20.4234998482374,-12.1406464752050;34.9662774645120,22.3048610747550;27.5135014076671,-11.8821136728163;43.3930560102998,29.1918291598582;11.6077007014000,-20.6506922893688;14.2726521436761,43.6692489761432;26.0464241886903,-9.68461191223183;28.5719086471357,-10.8625362969641;-44.8168664480278,-13.6630468269807;23.5832355674709,13.5178565205153;-0.595190155998191,32.6675264444015;-29.9910715366289,45.6368482533294;11.1109896755286,21.9724926010718;2.41096999999016,-30.8928020058105;-17.6380174262979,5.70411447112569;44.7963438180664,1.56617907096882;-20.6073071149438,-1.13858395595620;-20.9577988920251,5.42344400162102;-49.5887758676920,-6.17198415081061;-34.0672953155536,-23.4293882641728;42.0964373437748,2.08995994157947;16.0594842530402,-5.82742188618444;-24.1979673298498,20.0846357449426;14.1637955150501,-22.4093782451237;32.5019316440185,-47.7850742497659;5.65020748573521,-11.0558169220352;18.2860320074285,-13.5071921579294;-17.1338584251542,-0.289471368113610;79.8912249283554,-5.88289863046220;10.6167563438988,-21.6598424073464;-13.7120799496915,-25.7154131557099;29.4525761375705,-12.7340321868342;-52.3779403317386,48.4475929312710;-21.1053810203369,8.67400007274519;1.22993887326798,-3.70624692809957;-9.49856413179175,0.365690191879251;3.12900384491283,-0.904046456494743;7.50031956301589,12.3562905429823;6.43847488045511,39.2896929930343;30.9682913693970,-5.61260179380429;16.7208437458437,-8.93490027926457;9.16686338753494,56.7173561810963;0.0624559228070524,37.6697462339016;2.26330809713934,-31.5009505093967;-23.0049138108282,-41.5936241178010;-62.7614859944072,-28.5377598082390;-20.3656390340748,26.5074415703121;13.0862756695891,32.7324925017909;-14.8270753763793,-5.78908508095375;-36.7521730583284,9.86331038699916;30.7962679604583,-29.8559393603953;3.30373449393291,-10.5420304923620;-8.88117192704538,41.3303683202268;52.8999308566504,49.2318116154372;2.64158643963260,29.7777212516651;-31.9516412904338,66.0214783191805;25.7858271202722,-0.599436983789141;-33.1933459392193,-93.7843176189170;-21.9684124077570,-10.0769874165693;-46.2472363729114,-14.3156847131541;28.5206530919700,-37.9884661829570;-19.8272908012971,69.8206134424084;-60.3758844801787,-42.4986961801329;-48.0099240618389,43.2234111412034;36.9254540912872,-13.1099151080403;-5.68510756080214,-26.0976234853871;-8.11958271580063,13.3720867169582;-21.0633654435240,16.7354311467768;-57.1207020235893,35.5563977733588;-65.1929314913375,-21.9837655787721;-37.6217408807725,-20.6384038955951;84.2465567073162,27.1791826321299;39.8658260327592,-10.6410700792742;-26.7682286164832,-72.3620841457909;1.74228260500578,14.6987682407339;21.8314451872695,15.1545073222707;42.7734556804950,23.3053437107014;-52.3620474579486,-20.3070405291868;19.2066460686292,15.7282876188390;-28.1106773217216,43.0106924395391;4.34091817403331,-0.938947535803997;8.15815993778319,7.00469292746946;-8.95604207834383,-15.3998774409149;30.8017678895126,42.4660493858867;-17.2027808718314,-43.0309249568029;-21.9058944343869,7.63216437262147;-15.8982331214174,-87.8145268594438;-27.7880796216369,-62.1366554729360;-41.9872676071158,-37.0115089790813;-11.7876138344444,-18.6291455076347;-7.47108258146190,8.03099015819682;20.3031299554645,33.4991878115674;38.0367786645124,-45.9246778881033;-8.29756542801905,-18.7227382185443;-33.6772876877293,-8.13292522732060;1.23339911855664,24.2129095366567;19.4308341367927,-30.5938654997904;6.79504332625115,-12.8844642712938;4.09955943436103,-20.5529136861469;11.6474041405598,-10.2871769777538;-32.8559493774495,5.71941024997113;-13.3710644186996,-0.402235293952540;-55.3649370062477,9.90949896419729;10.3270944663458,-29.8206623734780;4.22237250760553,-15.4172531344176;-15.4388166937508,-38.9411634802937;-30.2422972307137,71.4956633189874;-12.9295495050203,-20.4110897033136;-48.0054796021967,-9.08675732421978;-25.6056200193537,3.17644033581957;30.6981662616174,61.6688203564539;-45.2662334936500,27.7915162166928;14.4139129010152,21.0677813690493;-53.2017685177607,-35.7644445241302;24.1028061148554,-5.04209787159278;40.7333655228055,-41.1553973407627;-43.5388328453299,10.8684050043691;-30.4708782776919,-7.55038729329319;20.0091647944412,-31.2798983911486;-1.19761713513697,34.5151579892012;-52.1267782097328,-54.7999948864971;-3.43666069424264,-26.5011615898042;-2.03310965759943,25.9285263561512;-26.0608455261549,-1.94358186102191;22.2739611789588,16.2564688893720;10.3975189569990,-50.9892153592224;-64.2056486613328,7.47116060246074;-15.5306111774140,-75.4292639210629;-14.4846452736577,50.1733276192943;0.0536610508167438,-3.27928990065061;-39.0545284067751,17.6636910104571;60.8120997091226,59.6641132793492;-4.18651394222449,33.4671448130509;-8.25243891799725,11.4486964692483;-25.9357479933522,-30.2822733916141;-27.3681458591677,0.342036135988558;6.97838101085754,8.20864206293599;3.03038466844881,-58.2632778760971;16.8993606770075,27.9108422231432;-27.0306341473338,-16.4765235366297;12.3646480910480,-27.9789983458528;-41.4985406489430,-13.0317554805855;-37.3791894534236,-8.50333619541164;-11.8982142980850,7.92441211996077;-9.72327330637509,12.1774956717125;15.9151700148394,20.6586769292605;41.4517412948654,-33.8120618698675;-39.2097412558798,-35.0917718016543;-1.36102370170649,-23.6649017506674;33.8944529438942,-33.8691869760874;-11.5688556677587,6.90628898547454;-0.278997796545284,-40.2141298570031;-13.7583283899933,13.1495187767439;-2.55425370337439,18.7363075473572;-39.4201451724125,32.9554924738448;36.7914506136300,-25.3543367232876;-12.7478218817958,47.9692398155069;10.2153628006544,9.87314562341864;-10.5614702168624,-13.0679362604975;20.8754008242970,6.54992052454898;-16.0458783309429,-40.5324064255838;30.3903700568314,9.34371987004970;-5.73837021567895,-25.6544990836216;15.4677589505125,-5.46693028001366;-47.3470681950565,-26.7624365219556;55.1855894325610,56.7414574276919;4.95842686431410,-35.6265373056285;29.7658408895663,6.11363001016659;-10.2831888009040,-22.1198355665407;10.0974051267114,26.9308351287914;-15.7852653064450,2.38949940621357;-50.5623081232901,9.59402907412139;-39.1366095708553,-11.7415086290372;12.7641711957722,-45.7962691570206;15.6936239614246,12.2595525827837;-21.3232661826075,-65.2199146482455;20.0508832545707,35.9684970232014;-19.7384288284593,15.6196390009822;-15.1826405246133,11.8802271472769;-6.40511792295145,-13.1342969543437;-0.907888672104065,19.9790797942738;-3.62858905372617,27.5934815700635;-10.2941327496090,-65.8643234916195;5.14557929572198,-15.0513081657779;46.3680947983112,-24.3541482668530;-8.64616721191304,-21.8697002119886;42.0890073145846,0.606048851138131;-2.06520021899472,-30.0471840716136;-21.7210791340497,-9.25588737795911;-30.1012999580862,-1.07385072967672;44.0154506521947,27.1629656743690;11.8497051934589,24.2944668413671;-9.16626772673761,-0.594061241792559;-3.30673632578662,47.9350979629852;38.6763561458939,-52.8725841883569;30.9713154780136,-29.3188547199508;25.2369382014317,-30.9360615257859;42.4411313477873,13.3429221299133;-5.93919430230613,5.47803671824044;42.5121640232097,4.00601476069030];

b1 = [-1.41578459326034;-2.82092899987627;59.0356966809787;1.95735210329088;42.1258073093999;-21.1530754048030;15.4887107360881;-22.5055757016112;-23.9141862595946;6.77577465043399;17.2713168247443;47.1535459988866;-4.05222361500415;-30.6779726437095;15.3284894597964;-34.3909321412271;-8.70067953202571;-23.3627992414523;74.1242182039947;-21.5239905543141;-10.9298722059985;-51.9492934875252;-27.2471598532389;12.1143508112316;5.00848134268408;26.3939169589766;-104.155929798891;12.3899988965416;11.9636053325023;9.64313160063835;10.3060984564103;43.7000100807576;24.0940727796438;-44.7171008926868;8.48733837560666;4.25341308629630;-3.41372838609989;14.8072353627375;-30.4192646449427;26.6454170258175;46.3646798774843;14.2951460454036;58.0530577872424;29.8535893965994;-33.3061851493480;10.9892834656023;-4.22404781851013;21.7713188748972;34.6226474451749;10.2209634387021;37.3391094119463;1.86788778897794;-0.0675788412840398;31.5952788012748;-1.08664735238556;-71.7575513391381;-22.0171077937529;-90.9688223607547;-65.1801329203165;0.345227188031911;13.4609669627993;-25.2909110084123;12.8813606661656;-46.3553247124562;-7.75491942746051;-3.32590178054242;66.6987631406210;67.1743195714668;-47.1969891013201;-15.2496739518154;-13.6508730837599;-10.6327162176596;-19.8361167861285;-5.12484859920138;19.7730222969171;12.9849075909486;9.11013268021325;-43.7446090209168;-24.0542831410782;59.6651772834574;40.1085671984201;30.1480216516469;9.43938856462673;8.62921735161748;-17.4508913281396;-6.23645449465104;-13.7439416713560;17.4066161457330;15.2825001089904;-69.3634915394675;-34.8282598066542;-19.6826353398984;-48.4201486104626;23.3577371607718;32.5573605800370;-34.0216935480320;22.8322536855958;-10.1916274294615;11.9593405472661;-25.3207892533329;-3.00798249768846;-62.2087954345408;38.0536952897753;28.0460446771128;-37.0358963442909;-17.8332312771059;15.9890882227126;27.7278823639036;30.5981806364709;40.7795949146865;34.7228182322281;42.5785109986169;-0.630592476975875;-20.7710667172622;-40.1921021072622;-3.61572592929096;-7.61470696573761;17.8589972981944;3.22487611554499;-33.3665328060293;12.5560899208583;-30.2935877783020;22.6285888324673;-6.67658307047059;-6.47269011107394;15.7204223516952;37.2884882430551;26.2771404082753;-4.96850196750291;-24.5253905894278;-39.7050478102623;-34.8076431126517;-5.93505171952133;-13.8168904414516;-39.0247371672724;16.6358385951829;9.60711649357348;-76.0658763351351;-38.3857342736788;-22.4611008799548;5.28931074732505;-54.0666547341457;-32.5984090826175;-13.7375886988174;5.96139526036785;39.8299243481843;-9.15029835353282;-41.3266663097817;26.8207034186434;24.4347571225535;75.9668101941652;63.8857816040636;-5.77776135875465;-24.9470618846799;-6.07008601903334;20.8528345247637;-10.7408702379504;-21.3939514632402;24.4114793368348;-77.3687770040019;42.0571360679851;-54.1497557564421;50.6871467941023;-8.21127804440150;45.1566721241092;-4.24218205742433;34.4380526628994;22.8225222233971;-20.5893985868623;-9.73799757160003;-7.54281291112240;36.7162712197463;25.9228625160238;10.3135578357506;75.7170988255583;-40.2141742332116;-16.0979771995405;32.5525892665365;-30.9485056936810;-31.5508009507046;-4.31144487579056;-17.0906692828626;10.3956563503828;17.6945196647626;-7.82950750936181;0.0183156023018338;4.09366348186716;-10.7440800459784;-13.1456759009841;19.8611883709011;31.1208206462208;27.1727378870761;-30.8133416353591;-12.1245994625966;-49.3926631775727;-65.3407088204555;21.2487016779601;11.9526212592363;32.4166611907064;-28.5588790866186];

W_out = [-0.00160412117838860,-0.00347244786098599,0.00174704566597939,0.00170245300978422,0.00174703169614077,0.0124382656067610,0.00174377206712961,-0.0177219044417143,-0.00174960028380156,0.00174947269260883,0.00174914766103029,0.00174944940954447,-0.00350552378222346,-0.00175005383789539,0.0176787991076708,0.00949191488325596,-0.00174970831722021,-0.00174971017986536,0.00174970459192991,-0.00174971017986536,0.00949191255494952,-0.00174970645457506,-0.00174963567405939,0.0147557985037565,-0.0124501967802644,0.00174970645457506,-0.00174970366060734,-0.00949199683964253,0.00174773298203945,-0.00941842608153820,0.00351360812783241,0.00174970366060734,0.0177132878452539,-0.00174970272928476,0.00174978282302618,-0.00948831159621477,-0.00550067611038685,0.00174971390515566,0.0124527690932155,0.00174970552325249,0.00174970645457506,0.00174971390515566,0.00174970366060734,0.00862028170377016,-0.00174970366060734,0.00351076480001211,0.0108524486422539,0.00174970645457506,0.00174971390515566,-0.00949196517467499,0.00174965709447861,-0.0123119913041592,0.00433791172690690,0.00174970924854279,-0.00478811934590340,-0.00174751412123442,0.00953402370214462,-0.00174970366060734,-0.00174970552325249,-0.00226417463272810,0.0147666260600090,0.0124528193846345,0.00351076480001211,-0.00124979484826326,0.00949188694357872,-0.00171803869307041,0.00174971390515566,0.00174970179796219,-0.00174971297383308,-0.00174970552325249,-0.00174971297383308,-0.00351076200604439,0.00949191581457853,-0.00174788013100624,0.00174970552325249,0.00174971017986536,0.00174971017986536,-0.00174971111118793,0.0254530170932412,0.00174970738589764,0.00174970924854279,0.00174971017986536,-0.00565755786374211,0.00174969900399446,-0.00174971111118793,-0.00781722366809845,-0.00174969993531704,0.00351075921207666,0.00351076340302825,-0.00174971576780081,-0.00174970552325249,-0.00464207003824413,-0.00174971297383308,-0.0254436172544956,-0.00750656193122268,-0.00174971483647823,0.0147523637861013,-0.00177515484392643,-0.0124478079378605,-0.00174970645457506,-0.0140285631641746,-0.00174970552325249,-0.00949194561690092,0.0121902357786894,-0.00174970831722021,-0.00174970366060734,0.0177132869139314,-0.0254554245620966,-0.00949191302061081,0.00174971669912338,0.00174971297383308,0.0178727954626083,-0.00390782393515110,-0.00174970366060734,-0.00174971111118793,-0.0176253151148558,-0.0144038489088416,-0.00949191674590111,-0.0123965535312891,0.000425099628046155,0.00351076433435082,-0.00174971204251051,0.00174970645457506,-0.00174971856176853,-0.00351074617356062,-0.0124528212472796,-0.00949191488325596,-0.0124528165906668,0.0124504659324884,-0.00174970552325249,-0.00174970366060734,-0.00351076107472181,0.0124526293948293,-0.00141679309308529,-0.00174970086663961,-0.00949190743267536,0.00174970831722021,-0.00174970924854279,0.0254555093124509,-0.00174971111118793,-0.0124521106481552,-0.00174970552325249,-0.00174971111118793,-0.00174923427402973,0.0177100962027907,0.00174970552325249,-0.0121920104138553,-0.00174971017986536,0.00106083974242210,0.0147523842751980,0.00174971111118793,0.00174970924854279,-0.0147525146603584,-0.00174963753670454,-0.0147526487708092,0.0147257074713707,0.0124528184533119,0.00138141121715307,-0.00581884616985917,-0.00174970831722021,-0.0233563655056059,-0.00174973625689745,0.00174970924854279,0.00966081954538822,-0.00897687207907438,-0.00351246772333980,0.00889056641608477,0.00174970738589764,-0.00174971017986536,-0.00145872961729765,-0.00174751691520214,-0.00950880162417889,-0.00949191581457853,-0.0124528203159571,0.00174970924854279,-0.00174970552325249,-0.00351483281701803,0.00174970924854279,-0.00174970831722021,-0.00174970552325249,0.0124499499797821,0.0124527756124735,-0.000751228304579854,0.00161213148385286,0.00949188927188516,0.00432793144136667,0.00174021162092686,-0.00174970831722021,-0.00174970645457506,-0.00949191534891725,0.00174970645457506,0.00174970552325249,-0.00174970645457506,0.0124528231099248,-0.00174970738589764,-0.00174970738589764,0.0147524178028107,0.00174970645457506,0.00174971111118793,0.00949191674590111];

output = W_out*tanh(W_in*[input_a input_b]' + b1);

end
